simulink model "FinalProject_Harness"  (R2023a)
settings: Solver=ode1be  StartTime=0.0  StopTime=10  RelTol=1e-3
settings Model: Creator=mrrom  LastModifiedBy=mrrom

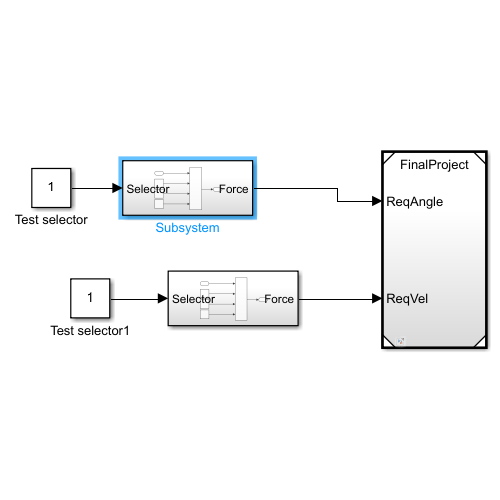
[thumbnail: Simulink's stored preview of the top-level diagram]
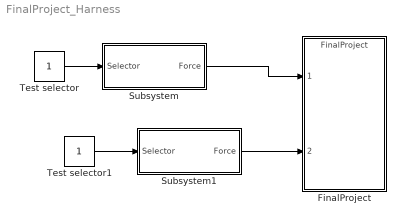
== system FinalProject_Harness ==
  FinalProject : ModelReference  ModelNameDialog=FinalProject  SimulationMode=Normal  ModelReferenceVersion=1.11
  Subsystem : Subsystem
  Subsystem1 : Subsystem
  Test selector : Constant
  Test selector1 : Constant
  wires:
  Test selector/1 -> Subsystem/1(Selector)
  Test selector1/1 -> Subsystem1/1(Selector)
  Subsystem1/1(Force) -> FinalProject/2
  Subsystem/1(Force) -> FinalProject/1

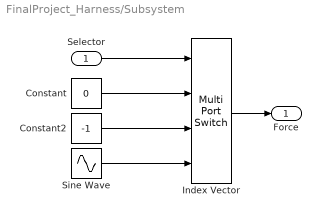
== system FinalProject_Harness/Subsystem ==
  Selector : Inport
  Constant : Constant  Value=0
  Constant2 : Constant  Value=-1
  Index Vector : MultiPortSwitch  SaturateOnIntegerOverflow=off  InputSameDT=off
  Sine Wave : Sin  Frequency=10  SampleTime=0
  Force : Outport
  wires:
  Index Vector/1 -> Force/1
  Selector/1 -> Index Vector/1
  Constant/1 -> Index Vector/2
  Constant2/1 -> Index Vector/3
  Sine Wave/1 -> Index Vector/4

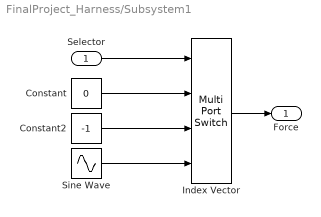
== system FinalProject_Harness/Subsystem1 ==
  Selector : Inport
  Constant : Constant  Value=0
  Constant2 : Constant  Value=-1
  Index Vector : MultiPortSwitch  SaturateOnIntegerOverflow=off  InputSameDT=off
  Sine Wave : Sin  Frequency=10  SampleTime=0
  Force : Outport
  wires:
  Index Vector/1 -> Force/1
  Selector/1 -> Index Vector/1
  Constant/1 -> Index Vector/2
  Constant2/1 -> Index Vector/3
  Sine Wave/1 -> Index Vector/4
